simulink model "ModelSFwithObs"  (R2019b)
settings: Solver=VariableStepAuto  StartTime=0.0  StopTime=1500  RelTol=1e-3
values from neighbouring files (symbols this model uses):
  A = [0 -th2 0 th4 0; 0 -1/th3 1/th3 0 0; 0 0 -1/th3 0 0 ... (first row only)    [AugmentedRev1.m]
  B = [0 0; 0 0; 1/th3 0; 0 0; 0 1/th5]    [AugmentedRev1.m]
  Bc = [th1; 0; 0; 0; 0]    [AugmentedRev1.m]
  C = [1 0 0 0 0]    [AugmentedRev1.m]
  Fin = k*[1/th2 -th3 -th3 (th5*th4)/(th2) (th5*th4)/(th2)]    [AugmentedRev1.m]
  L = [0.5; 0; 0.0; 0; 0]    [AugmentedRev1.m]
  th1 = 0.85    [AugmentedRev1.m]
  th2 = 50    [AugmentedRev1.m]
  th3 = 60    [AugmentedRev1.m]
  x0 = [110; th1/th2; th1/th2; 0; 0]    [AugmentedRev1.m]
settings Model: Creator=akshita_jain  LastModifiedBy=akshita_jain

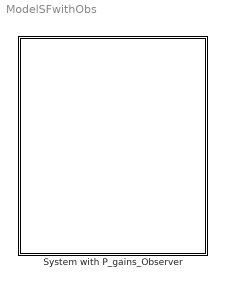
== system ModelSFwithObs ==
  System with P_gains_Observer : Subsystem

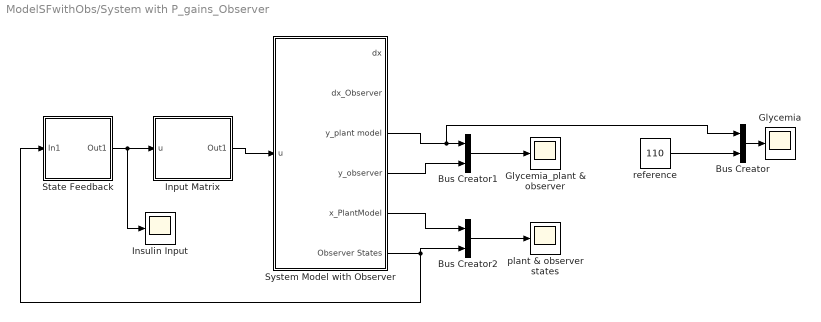
== system ModelSFwithObs/System with P_gains_Observer ==
  Bus Creator : BusCreator  Inputs=2
  Bus Creator1 : BusCreator  Inputs=2
  Bus Creator2 : BusCreator  Inputs=2
  Glycemia : Scope
  Glycemia_plant & observer : Scope
  Input Matrix : Subsystem
  Insulin Input : Scope
  "State Feedback " : Subsystem
  System Model with Observer : Subsystem
  plant & observer states : Scope
  reference : Constant  Value=110
  wires:
  reference/1 -> Bus Creator/2
  Bus Creator/1 -> Glycemia/1
  Input Matrix/1(Out1) -> System Model with Observer/1(u)
  Bus Creator1/1 -> Glycemia_plant & observer/1
  Bus Creator2/1 -> plant & observer states/1
  "State Feedback "/1(Out1) -> Insulin Input/1, Input Matrix/1(u)
  System Model with Observer/5(x_PlantModel) -> Bus Creator2/1
  System Model with Observer/6(Observer States) -> "State Feedback "/1(In1), Bus Creator2/2
  System Model with Observer/3(y_plant model) -> Bus Creator/1, Bus Creator1/1
  System Model with Observer/4(y_observer) -> Bus Creator1/2

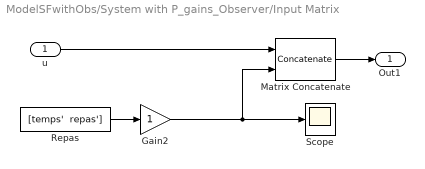
== system ModelSFwithObs/System with P_gains_Observer/Input Matrix ==
  u : Inport
  Gain2 : Gain
  Matrix Concatenate : Concatenate  ConcatenateDimension=2
  Repas : FromWorkspace  VariableName="[temps'  repas']"  SampleTime=0
  Scope : Scope
  Out1 : Outport
  wires:
  u/1 -> Matrix Concatenate/1
  Matrix Concatenate/1 -> Out1/1
  Gain2/1 -> Scope/1, Matrix Concatenate/2
  Repas/1 -> Gain2/1

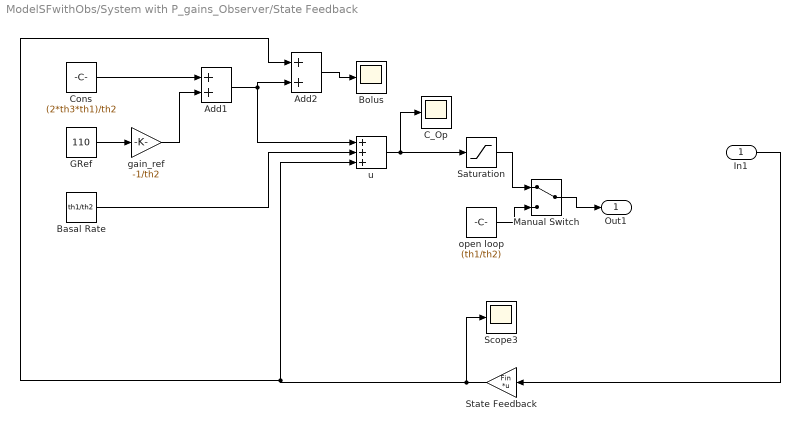
== system ModelSFwithObs/System with P_gains_Observer/State Feedback  ==
  In1 : Inport
  Add1 : Sum
  Add2 : Sum
  Basal Rate : Constant  Value=th1/th2  VectorParams1D=off
  Bolus : Scope
  C_Op : Scope
  Cons : Constant  Value=(2*th3*th1)/th2  VectorParams1D=off
  GRef : Constant  Value=110
  Manual Switch : ManualSwitch
  Saturation : Saturate  UpperLimit=2  LowerLimit=0
  Scope3 : Scope
  State Feedback : Gain  Gain=Fin  Multiplication=Matrix(K*u)
  gain_ref : Gain  Gain=-1/th2
  open loop : Constant  Value=(th1/th2)
  "u " : Sum  Inputs=+++
  Out1 : Outport
  wires:
  Manual Switch/1 -> Out1/1
  State Feedback/1 -> "u "/3, Add2/1, Scope3/1
  In1/1 -> State Feedback/1
  gain_ref/1 -> Add1/2
  Add2/1 -> Bolus/1
  Basal Rate/1 -> "u "/2
  "u "/1 -> C_Op/1, Saturation/1
  open loop/1 -> Manual Switch/2
  GRef/1 -> gain_ref/1
  Saturation/1 -> Manual Switch/1
  Add1/1 -> "u "/1, Add2/2
  Cons/1 -> Add1/1

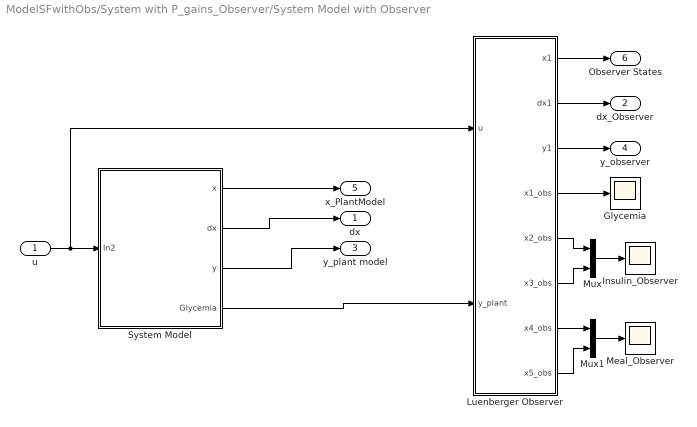
== system ModelSFwithObs/System with P_gains_Observer/System Model with Observer ==
  u : Inport
  Glycemia : Scope
  Insulin_Observer : Scope
  Luenberger Observer : Subsystem
  Meal_Observer : Scope
  Mux : Mux  Inputs=2
  Mux1 : Mux  Inputs=2
  System Model : Subsystem
  dx : Outport
  dx_Observer : Outport  Port=2
  y_plant model : Outport  Port=3
  y_observer : Outport  Port=4
  x_PlantModel : Outport  Port=5
  Observer States : Outport  Port=6
  wires:
  Luenberger Observer/1(x1) -> Observer States/1
  Luenberger Observer/2(dx1) -> dx_Observer/1
  Luenberger Observer/3(y1) -> y_observer/1
  u/1 -> Luenberger Observer/1(u), System Model/1(In2)
  System Model/1(x) -> x_PlantModel/1
  System Model/2(dx) -> dx/1
  System Model/3(y) -> y_plant model/1
  System Model/4(Glycemia) -> Luenberger Observer/2("y_plant ")
  Luenberger Observer/4(x1_obs) -> Glycemia/1
  Luenberger Observer/5(x2_obs) -> Mux/1
  Luenberger Observer/6(x3_obs) -> Mux/2
  Mux/1 -> Insulin_Observer/1
  Luenberger Observer/7(x4_obs) -> Mux1/1
  Luenberger Observer/8(x5_obs) -> Mux1/2
  Mux1/1 -> Meal_Observer/1

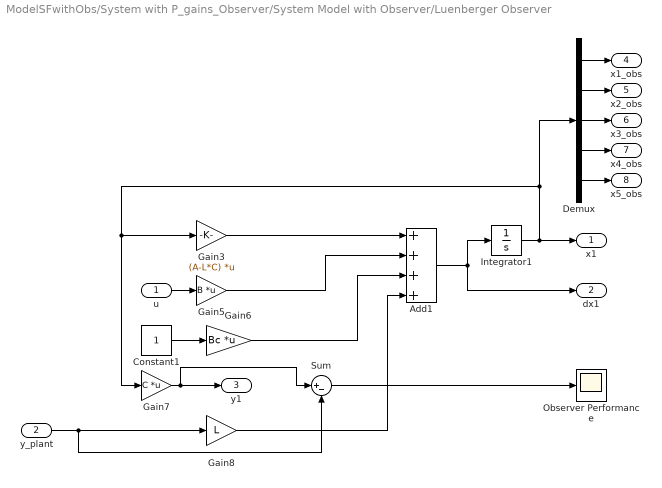
== system ModelSFwithObs/System with P_gains_Observer/System Model with Observer/Luenberger Observer ==
  u : Inport
  "y_plant " : Inport  Port=2
  Add1 : Sum  Inputs=4
  Constant1 : Constant
  Demux : Demux  Outputs=5
  Gain3 : Gain  Gain=(A-L*C)  Multiplication=Matrix(K*u)
  Gain5 : Gain  Gain=B  Multiplication=Matrix(K*u)
  Gain6 : Gain  Gain=Bc  Multiplication=Matrix(K*u)
  Gain7 : Gain  Gain=C  Multiplication=Matrix(K*u)
  Gain8 : Gain  Gain=L
  Integrator1 : Integrator  InitialCondition=[115; th1/th2; th1/th2; 0; 0]  ZeroCross=off
  Observer Performance : Scope
  Sum : Sum  Inputs=|+-
  x1 : Outport
  dx1 : Outport  Port=2
  y1 : Outport  Port=3
  x1_obs : Outport  Port=4
  x2_obs : Outport  Port=5
  x3_obs : Outport  Port=6
  x4_obs : Outport  Port=7
  x5_obs : Outport  Port=8
  wires:
  u/1 -> Gain5/1
  Sum/1 -> Observer Performance/1
  "y_plant "/1 -> Sum/2, Gain8/1
  Add1/1 -> dx1/1, Integrator1/1
  Gain6/1 -> Add1/3
  Constant1/1 -> Gain6/1
  Integrator1/1 -> x1/1, Gain3/1, Gain7/1, Demux/1
  Gain3/1 -> Add1/1
  Gain5/1 -> Add1/2
  Gain8/1 -> Add1/4
  Gain7/1 -> y1/1, Sum/1
  Demux/1 -> x1_obs/1
  Demux/2 -> x2_obs/1
  Demux/3 -> x3_obs/1
  Demux/4 -> x4_obs/1
  Demux/5 -> x5_obs/1

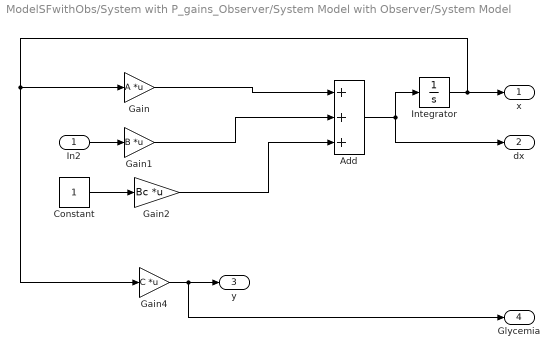
== system ModelSFwithObs/System with P_gains_Observer/System Model with Observer/System Model ==
  In2 : Inport
  Add : Sum  Inputs=3
  Constant : Constant
  Gain : Gain  Gain=A  Multiplication=Matrix(K*u)
  Gain1 : Gain  Gain=B  Multiplication=Matrix(K*u)
  Gain2 : Gain  Gain=Bc  Multiplication=Matrix(K*u)
  Gain4 : Gain  Gain=C  Multiplication=Matrix(K*u)
  Integrator : Integrator  InitialCondition=x0  ZeroCross=off
  x : Outport
  dx : Outport  Port=2
  y : Outport  Port=3
  Glycemia : Outport  Port=4
  wires:
  Gain2/1 -> Add/3
  Gain1/1 -> Add/2
  Gain4/1 -> Glycemia/1, y/1
  Gain/1 -> Add/1
  Constant/1 -> Gain2/1
  In2/1 -> Gain1/1
  Add/1 -> dx/1, Integrator/1
  Integrator/1 -> x/1, Gain/1, Gain4/1
